simulink model "Final_Project_Simulink_Model"  (R2025b)
settings: Solver=FixedStepAuto  StartTime=0.0  StopTime=60.0  RelTol=1e-3  EnableMultiTasking=on
libraries: arduinolib x3, arduinosensorlib x1, simulink x1
settings Model: ExtModeTrigDuration=2  Creator=Phill  LastModifiedBy=Phill
settings SolverCC: AutoInsertRateTranBlk=on
settings OptimizationCC: EnhancedBackFolding=on  PassReuseOutputArgsAs=Individual arguments  ZeroExternalMemoryAtStartup=off  ZeroInternalMemoryAtStartup=off  MaxStackSize=64  OptimizeBlockOrder=speed  DifferentSizesBufferReuse=on  OptimizationCustomize=off  EfficientTunableParamExpr=on
settings DebuggingCC: ParameterTunabilityLossMsg=error
settings HardwareCC: ProdBitPerInt=16.0  ProdBitPerPointer=16.0  ProdBitPerSizeT=16.0  ProdBitPerPtrDiffT=16.0  ProdLargestAtomicFloat=None  ProdWordSize=8.0  ProdHWDeviceType=Atmel->AVR
settings SFSimCC: MATLABDynamicMemAlloc=off
settings RTWCC: SystemTargetFile=ert.tlc  HardwareBoard=Arduino Uno  TemplateMakefile=ert_default_tmf  Toolchain=Arduino AVR  BuildConfiguration=Faster Runs  Description=Embedded Coder
settings CodeAppCC: ForceParamTrailComments=on  IgnoreCustomStorageClasses=off  OperatorAnnotations=on  SimulinkDataObjDesc=on  SFDataObjDesc=on  InsertBlockDesc=on
settings ERTTargetCC: ExtModeTransport=3.0  ExtModeStaticAlloc=on  ExtModeAutomaticAllocSize=off  ExtModeStaticAllocSize=250.0  ExtModeMexFile=ext_xcp  ExtModeIntrfLevel=Level2 - Open  InlinedParameterPlacement=Hierarchical  SupportContinuousTime=on  SupportVariableSizeSignals=on

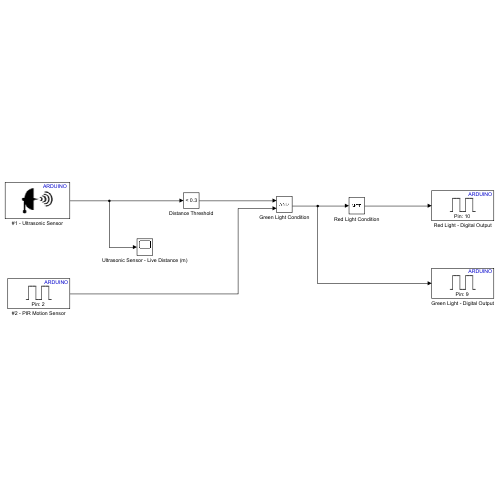
[thumbnail: Simulink's stored preview of the top-level diagram]
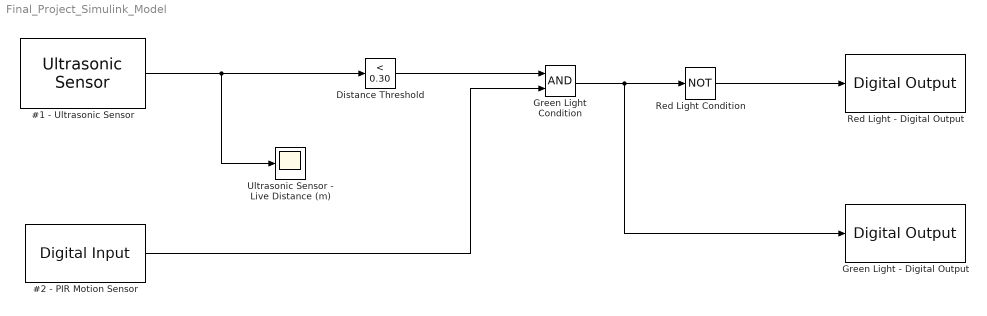
== system Final_Project_Simulink_Model ==
  #1 - Ultrasonic Sensor : arduinosensorlib/Ultrasonic Sensor  NumSignalPins=2  TrigPin=11  EchoPin=12  SignalPin=3  SampleTime_=0.1  blockPlatform=ARDUINO
  #2 - PIR Motion Sensor : arduinolib/Digital Input  pinNumber=2  mode=Default  Direction=input  SampleTime=0.1  blockPlatform=arduino
  Distance Threshold : simulink/Logic and Bit Operations/Compare To Constant  relop=<  const=0.30  OutDataTypeStr=boolean
  Green Light - Digital Output : arduinolib/Digital Output  pinNumber=9  Direction=output  blockPlatform=arduino
  Green Light Condition : Logic  AllPortsSameDT=off  OutDataTypeStr=boolean
  Red Light - Digital Output : arduinolib/Digital Output  pinNumber=10  Direction=output  blockPlatform=arduino
  Red Light Condition : Logic  Operator=NOT  AllPortsSameDT=off  OutDataTypeStr=boolean
  Ultrasonic Sensor - Live Distance (m) : Scope
      settings: ActiveDisplayYMinimum=0  ActiveDisplayYMaximum=2  YLabel=Distance (meters)
  wires:
  Distance Threshold/1 -> Green Light Condition/1
  #2 - PIR Motion Sensor/1 -> Green Light Condition/2
  Green Light Condition/1 -> Green Light - Digital Output/1, Red Light Condition/1
  Red Light Condition/1 -> Red Light - Digital Output/1
  #1 - Ultrasonic Sensor/1 -> Ultrasonic Sensor - Live Distance (m)/1, Distance Threshold/1
